simulink model "black_box"  (R2024b)
settings: Solver=ode1  StartTime=0.0  StopTime=Tobs  FixedStep=Ts  RelTol=1e-3
values from neighbouring files (symbols this model uses):
  delta_t = 10E-6    (= 1e-05)    [main_SVD.m]    (also in main_scan_FD.m)
  f0 = 50    [main_SVD.m]    (also in main_scan_FD.m)
  Id_ss = 0    [main_scan_FD.m]
  Ipeak = Sbase/Vpeak    [main_scan_FD.m]
  Iq_ss = 0    [main_scan_FD.m]
  P_finalvalue = 0.486    [main_scan_FD.m]    (also in main_ss_composite.m = 0.05)
  P_step_time = 1.5    [main_scan_FD.m]    (also in main_ss_composite.m = 10)
  phi = 0 * pi / 180    (= 0)    [main_SVD.m]
  signal_type = 1    [main_scan_FD.m]
  Ts = delta_t    (= 1e-05)    [main_scan_FD.m]
  V_finalvalue = 0.99    [main_ss_composite.m]
  V_step_time = 100    [main_scan_FD.m]    (also in main_ss_composite.m = 10)
  Vd_ss = 0    [main_scan_FD.m]
  Vpeak = (Vbase/sqrt(3))*sqrt(2)    [main_scan_FD.m]
  Vq_ss = 0    [main_scan_FD.m]
undefined symbols (not defined in the file or in its folder): C_dc, C_filt, dist_time, dist_value_0, dist_value_a, dist_value_b, dist_value_c, dist_value_d, dist_value_n, dist_value_p, dist_value_q, f_base, fd, I_charge, Iss_type, ki_inner_pu, ki_outer_P_pu, ki_outer_V_pu, ki_pll, kp_inner_pu, kp_outer_P_pu, kp_outer_V_pu, kp_pll, L, L_base, L_grid, L_vsc, omega_b, P_base, R_grid, R_vsc, Rsource, t_charge, V_base, V_dc, Vss_type
libraries: spsThreePhaseVIMeasurementLib x19, spsControlledVoltageSourceLib x15, spsControlledCurrentSourceLib x14, slpidlib x5, spsThreePhaseSeriesRLCBranchLib x4, spsabctodq0Lib x4, spsGroundLib x3, eeGeneralControl x1, spsLeadLagFilterLib x1, spsParallelRLCBranchLib x1, spsPLL3phLib x1, spsThreePhaseSourceLib x1
(part 3 of 3)

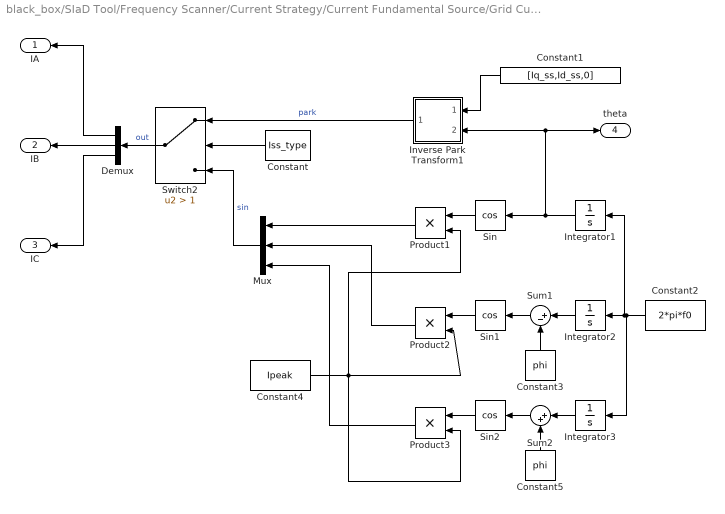
== system black_box/SIaD Tool/Frequency Scanner/Current Strategy/Current Fundamental Source/Grid Currents1 ==
  Constant : Constant  Value=Iss_type
  Constant1 : Constant  Value=[Iq_ss,Id_ss,0]  SampleTime=delta_t
  Constant2 : Constant  Value=2*pi*f0
  Constant3 : Constant  Value=phi
  Constant4 : Constant  Value=Ipeak
  Constant5 : Constant  Value=phi
  Demux : Demux  Outputs=3
  Integrator1 : Integrator  UpperSaturationLimit=1E100  LowerSaturationLimit=-1E100
  Integrator2 : Integrator  UpperSaturationLimit=1E100  LowerSaturationLimit=-1E100
  Integrator3 : Integrator  UpperSaturationLimit=1E100  LowerSaturationLimit=-1E100
  Inverse Park Transform1 : Subsystem
  Mux : Mux  Inputs=3
  Product1 : Product
  Product2 : Product
  Product3 : Product
  Sin : Trigonometry  Operator=cos
  Sin1 : Trigonometry  Operator=cos
  Sin2 : Trigonometry  Operator=cos
  Sum1 : Sum  Inputs=|+-
  Sum2 : Sum  Inputs=|++
  Switch2 : Switch  Criteria=u2 > Threshold  Threshold=1  SaturateOnIntegerOverflow=off  InputSameDT=off
  IA : Outport
  IB : Outport  Port=2
  IC : Outport  Port=3
  theta : Outport  Port=4
  wires:
  Constant1/1 -> Inverse Park Transform1/1(qd0)
  Demux/1 -> IA/1
  Demux/2 -> IB/1
  Demux/3 -> IC/1
  Product3/1 -> Mux/3
  Product1/1 -> Mux/1
  Sum1/1 -> Sin1/1
  Integrator2/1 -> Sum1/1
  Constant5/1 -> Sum2/2
  Integrator3/1 -> Sum2/1
  Sin/1 -> Product1/1
  Sin2/1 -> Product3/1
  Sin1/1 -> Product2/1
  Sum2/1 -> Sin2/1
  Constant2/1 -> Integrator1/1, Integrator2/1, Integrator3/1
  Integrator1/1 -> theta/1, Inverse Park Transform1/2(theta), Sin/1
  Constant4/1 -> Product2/2, Product1/2, Product3/2
  Product2/1 -> Mux/2
  Constant3/1 -> Sum1/2
  Switch2/1 -> Demux/1  "out"
  Inverse Park Transform1/1(ABC) -> Switch2/1  "park"
  Mux/1 -> Switch2/3  "sin"
  Constant/1 -> Switch2/2

== system black_box/SIaD Tool/Frequency Scanner/Current Strategy/pn0disturbance2/Multi-tone ==
  Clock : Clock
  Constant1 : Constant  Value=0
  From Workspace : FromWorkspace  VariableName=dist_value_0  SampleTime=delta_t  Interpolate=off  OutputAfterFinalValue=Holding final value
  From Workspace1 : FromWorkspace  VariableName=dist_value_p  SampleTime=delta_t  Interpolate=off  OutputAfterFinalValue=Holding final value
  From Workspace2 : FromWorkspace  VariableName=dist_value_n  SampleTime=delta_t  Interpolate=off  OutputAfterFinalValue=Holding final value
  Inverse Fortescue Transformation : Subsystem
  Mux : Mux  Inputs=3
  Switch1 : Switch  Criteria=u2 > Threshold  Threshold=dist_time  SaturateOnIntegerOverflow=off  InputSameDT=off
  Switch2 : Switch  Criteria=u2 > Threshold  Threshold=dist_time  SaturateOnIntegerOverflow=off  InputSameDT=off
  Switch3 : Switch  Criteria=u2 > Threshold  Threshold=dist_time  SaturateOnIntegerOverflow=off  InputSameDT=off
  ABC : Outport
  wires:
  Switch2/1 -> Mux/2
  From Workspace2/1 -> Switch3/1
  Constant1/1 -> Switch3/3, Switch2/3, Switch1/3
  From Workspace1/1 -> Switch2/1
  Switch3/1 -> Mux/3
  Clock/1 -> Switch1/2, Switch2/2, Switch3/2
  Switch1/1 -> Mux/1
  From Workspace/1 -> Switch1/1
  Mux/1 -> Inverse Fortescue Transformation/1(0PN)
  Inverse Fortescue Transformation/1(ABC) -> ABC/1

== system black_box/SIaD Tool/Frequency Scanner/Current Strategy/pn0disturbance2/Single-tone ==
  Constant1 : Constant  Value=2*pi*fd  SampleTime=delta_t
  Constant1111 : Constant  Value=0
  Constant222 : Constant  Value=dist_value_p
  Constant49 : Constant  Value=dist_value_0
  Constant50 : Constant  Value=dist_value_n
  Disturbance activator : Step  Time=dist_time  SampleTime=delta_t
  Integrator3 : Integrator
  Inverse Fortescue Transformation : Subsystem
  Math Function3 : Math
  Math Function4 : Math
  Math Function5 : Math
  Multiply2 : Gain
  Multiply3 : Gain
  Multiply4 : Gain
  Mux1 : Mux  Inputs=3
  Product{,4..5,8} (4 alike) : Product
  Real-Imag to Complex2 : RealImagToComplex
  Real-Imag to Complex3 : RealImagToComplex
  Real-Imag to Complex4 : RealImagToComplex
  ABC : Outport
  wires:
  Real-Imag to Complex3/1 -> Multiply2/1
  Math Function3/1 -> Product5/2
  Real-Imag to Complex2/1 -> Multiply3/1
  Inverse Fortescue Transformation/1(ABC) -> Product/2
  Disturbance activator/1 -> Product/1
  Product8/1 -> Mux1/2
  Integrator3/1 -> Real-Imag to Complex2/2, Real-Imag to Complex3/2, Real-Imag to Complex4/2
  Product/1 -> ABC/1
  Multiply2/1 -> Math Function4/1
  Real-Imag to Complex4/1 -> Multiply4/1
  Constant222/1 -> Product8/2
  Math Function5/1 -> Product4/2
  Constant49/1 -> Product4/1
  Mux1/1 -> Inverse Fortescue Transformation/1(0PN)
  Multiply3/1 -> Math Function3/1
  Multiply4/1 -> Math Function5/1
  Constant1/1 -> Integrator3/1
  Product4/1 -> Mux1/1
  Math Function4/1 -> Product8/1
  Constant1111/1 -> Real-Imag to Complex4/1, Real-Imag to Complex3/1, Real-Imag to Complex2/1
  Product5/1 -> Mux1/3
  Constant50/1 -> Product5/1

== system black_box/SIaD Tool/Frequency Scanner/Current Strategy/qd0disturbance2/Multi-tone ==
  In1 : Inport
  Clock1 : Clock
  Constant : Constant  Value=0
  From Workspace3 : FromWorkspace  VariableName=dist_value_q  SampleTime=delta_t  Interpolate=off  OutputAfterFinalValue=Holding final value
  From Workspace4 : FromWorkspace  VariableName=dist_value_d  SampleTime=delta_t  Interpolate=off  OutputAfterFinalValue=Holding final value
  Inverse Park Transform1 : Subsystem
  Mux3 : Mux  Inputs=3
  Switch : Switch  Criteria=u2 > Threshold  Threshold=dist_time  SaturateOnIntegerOverflow=off  InputSameDT=off
  Switch4 : Switch  Criteria=u2 > Threshold  Threshold=dist_time  SaturateOnIntegerOverflow=off  InputSameDT=off
  Vd : Constant  Value=0
  ABC : Outport
  wires:
  Inverse Park Transform1/1(ABC) -> ABC/1
  From Workspace3/1 -> Switch/1
  Clock1/1 -> Switch/2, Switch4/2
  Switch4/1 -> Mux3/2  "vd"
  Constant/1 -> Switch4/3, Switch/3
  Mux3/1 -> Inverse Park Transform1/1(qd0)
  Vd/1 -> Mux3/3
  From Workspace4/1 -> Switch4/1
  Switch/1 -> Mux3/1  "vq"
  In1/1 -> Inverse Park Transform1/2(theta)

== system black_box/SIaD Tool/Frequency Scanner/Current Strategy/qd0disturbance2/Single-tone ==
  note: qd disturbance
  In1 : Inport
  Constant18 : Constant  Value=dist_value_d
  Constant19 : Constant  Value=2*pi*fd
  Constant21 : Constant  Value=dist_value_q
  Cos : Trigonometry  Operator=cos
  Cos1 : Trigonometry  Operator=cos
  Disturbance activator : Step  Time=dist_time  Before=0.0  After=1.0  SampleTime=delta_t
  Integrator : Integrator
  Inverse Park Transform : Subsystem
  Mux23 : Mux  Inputs=3
  Product : Product
  Product4 : Product
  Product5 : Product
  V0 : Constant  Value=0
  ABC : Outport
  wires:
  Product/1 -> ABC/1
  Cos1/1 -> Product5/1
  Product4/1 -> Mux23/1
  Constant21/1 -> Product4/1
  Product5/1 -> Mux23/2
  Integrator/1 -> Cos/1, Cos1/1
  Cos/1 -> Product4/2
  Disturbance activator/1 -> Product/1
  Inverse Park Transform/1(ABC) -> Product/2
  Mux23/1 -> Inverse Park Transform/1(qd0)
  In1/1 -> Inverse Park Transform/2(theta)
  Constant18/1 -> Product5/2
  Constant19/1 -> Integrator/1
  V0/1 -> Mux23/3

== system black_box/SIaD Tool/Frequency Scanner/Voltage Strategy/ABCdisturbance/Multi-tone ==
  Clock : Clock
  Constant1 : Constant  Value=0
  From Workspace : FromWorkspace  VariableName=dist_value_a  SampleTime=delta_t  Interpolate=off  OutputAfterFinalValue=Holding final value
  From Workspace1 : FromWorkspace  VariableName=dist_value_b  SampleTime=delta_t  Interpolate=off  OutputAfterFinalValue=Holding final value
  From Workspace2 : FromWorkspace  VariableName=dist_value_c  SampleTime=delta_t  Interpolate=off  OutputAfterFinalValue=Holding final value
  Mux : Mux  Inputs=3
  Switch1 : Switch  Criteria=u2 > Threshold  Threshold=dist_time  SaturateOnIntegerOverflow=off  InputSameDT=off
  Switch2 : Switch  Criteria=u2 > Threshold  Threshold=dist_time  SaturateOnIntegerOverflow=off  InputSameDT=off
  Switch3 : Switch  Criteria=u2 > Threshold  Threshold=dist_time  SaturateOnIntegerOverflow=off  InputSameDT=off
  ABC : Outport
  wires:
  Switch2/1 -> Mux/2
  From Workspace2/1 -> Switch3/1
  Constant1/1 -> Switch3/3, Switch2/3, Switch1/3
  From Workspace1/1 -> Switch2/1
  Switch3/1 -> Mux/3
  Clock/1 -> Switch1/2, Switch2/2, Switch3/2
  Switch1/1 -> Mux/1
  From Workspace/1 -> Switch1/1
  Mux/1 -> ABC/1

== system black_box/SIaD Tool/Frequency Scanner/Voltage Strategy/ABCdisturbance/Single-tone ==
  note: ABC perturbance
  Constant10 : Constant  Value=phi
  Constant12 : Constant  Value=2*pi*fd  SampleTime=delta_t
  Constant9 : Constant  Value=phi
  Integrator5 : Integrator  UpperSaturationLimit=1E100  LowerSaturationLimit=-1E100
  Mux : Mux  Inputs=3
  Product1 : Product
  Product2 : Product
  Product3 : Product
  Sin : Trigonometry  Operator=cos
  Sin1 : Trigonometry  Operator=cos
  Sin2 : Trigonometry  Operator=cos
  Step1 : Step  Time=dist_time  After=dist_value_a  SampleTime=delta_t
  Step2 : Step  Time=dist_time  After=dist_value_b  SampleTime=delta_t
  Step3 : Step  Time=dist_time  After=dist_value_c  SampleTime=delta_t
  Sum6 : Sum  Inputs=|+-
  Sum7 : Sum  Inputs=|++
  ABC : Outport
  wires:
  Sin/1 -> Product1/1
  Sum7/1 -> Sin2/1
  Product1/1 -> Mux/1
  Integrator5/1 -> Sum7/1, Sin/1, Sum6/1
  Sin1/1 -> Product2/1
  Sin2/1 -> Product3/1
  Constant9/1 -> Sum6/2
  Constant10/1 -> Sum7/2
  Step3/1 -> Product3/2
  Step2/1 -> Product2/2
  Constant12/1 -> Integrator5/1
  Sum6/1 -> Sin1/1
  Step1/1 -> Product1/2
  Product2/1 -> Mux/2
  Product3/1 -> Mux/3
  Mux/1 -> ABC/1

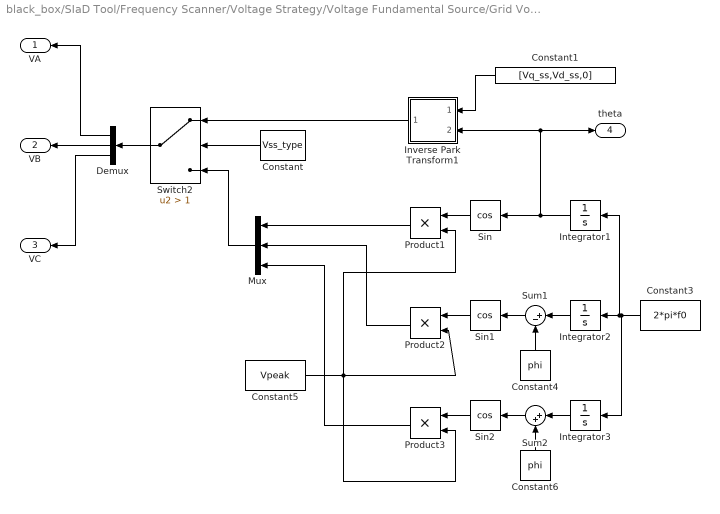
== system black_box/SIaD Tool/Frequency Scanner/Voltage Strategy/Voltage Fundamental Source/Grid Voltages ==
  Constant : Constant  Value=Vss_type
  Constant1 : Constant  Value=[Vq_ss,Vd_ss,0]  SampleTime=delta_t
  Constant3 : Constant  Value=2*pi*f0
  Constant4 : Constant  Value=phi
  Constant5 : Constant  Value=Vpeak
  Constant6 : Constant  Value=phi
  Demux : Demux  Outputs=3
  Integrator1 : Integrator  UpperSaturationLimit=1E100  LowerSaturationLimit=-1E100
  Integrator2 : Integrator  UpperSaturationLimit=1E100  LowerSaturationLimit=-1E100
  Integrator3 : Integrator  UpperSaturationLimit=1E100  LowerSaturationLimit=-1E100
  Inverse Park Transform1 : Subsystem
  Mux : Mux  Inputs=3
  Product1 : Product
  Product2 : Product
  Product3 : Product
  Sin : Trigonometry  Operator=cos
  Sin1 : Trigonometry  Operator=cos
  Sin2 : Trigonometry  Operator=cos
  Sum1 : Sum  Inputs=|+-
  Sum2 : Sum  Inputs=|++
  Switch2 : Switch  Criteria=u2 > Threshold  Threshold=1  SaturateOnIntegerOverflow=off  InputSameDT=off
  VA : Outport
  VB : Outport  Port=2
  VC : Outport  Port=3
  theta : Outport  Port=4
  wires:
  Demux/1 -> VA/1
  Demux/3 -> VC/1
  Demux/2 -> VB/1
  Constant5/1 -> Product2/2, Product1/2, Product3/2
  Mux/1 -> Switch2/3
  Product1/1 -> Mux/1
  Constant4/1 -> Sum1/2
  Integrator1/1 -> theta/1, Inverse Park Transform1/2(theta), Sin/1
  Product3/1 -> Mux/3
  Switch2/1 -> Demux/1
  Constant/1 -> Switch2/2
  Constant3/1 -> Integrator1/1, Integrator2/1, Integrator3/1
  Inverse Park Transform1/1(ABC) -> Switch2/1
  Sin1/1 -> Product2/1
  Integrator3/1 -> Sum2/1
  Integrator2/1 -> Sum1/1
  Sin2/1 -> Product3/1
  Constant1/1 -> Inverse Park Transform1/1(qd0)
  Sum2/1 -> Sin2/1
  Product2/1 -> Mux/2
  Constant6/1 -> Sum2/2
  Sin/1 -> Product1/1
  Sum1/1 -> Sin1/1

== system black_box/SIaD Tool/Frequency Scanner/Voltage Strategy/pn0disturbance/Multi-tone ==
  Clock : Clock
  Constant1 : Constant  Value=0
  From Workspace : FromWorkspace  VariableName=dist_value_0  SampleTime=delta_t  Interpolate=off  OutputAfterFinalValue=Holding final value
  From Workspace1 : FromWorkspace  VariableName=dist_value_p  SampleTime=delta_t  Interpolate=off  OutputAfterFinalValue=Holding final value
  From Workspace2 : FromWorkspace  VariableName=dist_value_n  SampleTime=delta_t  Interpolate=off  OutputAfterFinalValue=Holding final value
  Inverse Fortescue Transformation : Subsystem
  Mux : Mux  Inputs=3
  Switch1 : Switch  Criteria=u2 > Threshold  Threshold=dist_time  SaturateOnIntegerOverflow=off  InputSameDT=off
  Switch2 : Switch  Criteria=u2 > Threshold  Threshold=dist_time  SaturateOnIntegerOverflow=off  InputSameDT=off
  Switch3 : Switch  Criteria=u2 > Threshold  Threshold=dist_time  SaturateOnIntegerOverflow=off  InputSameDT=off
  ABC : Outport
  wires:
  Switch2/1 -> Mux/2
  From Workspace2/1 -> Switch3/1
  Constant1/1 -> Switch3/3, Switch2/3, Switch1/3
  From Workspace1/1 -> Switch2/1
  Switch3/1 -> Mux/3
  Clock/1 -> Switch1/2, Switch2/2, Switch3/2
  Switch1/1 -> Mux/1
  From Workspace/1 -> Switch1/1
  Mux/1 -> Inverse Fortescue Transformation/1(0PN)
  Inverse Fortescue Transformation/1(ABC) -> ABC/1

== system black_box/SIaD Tool/Frequency Scanner/Voltage Strategy/pn0disturbance/Single-tone ==
  Constant1 : Constant  Value=2*pi*fd  SampleTime=delta_t
  Constant1111 : Constant  Value=0
  Constant222 : Constant  Value=dist_value_p
  Constant49 : Constant  Value=dist_value_0
  Constant50 : Constant  Value=dist_value_n
  Disturbance activator : Step  Time=dist_time  SampleTime=delta_t
  Integrator3 : Integrator
  Inverse Fortescue Transformation : Subsystem
  Math Function3 : Math
  Math Function4 : Math
  Math Function5 : Math
  Multiply2 : Gain
  Multiply3 : Gain
  Multiply4 : Gain
  Mux1 : Mux  Inputs=3
  Product{,4..5,8} (4 alike) : Product
  Real-Imag to Complex2 : RealImagToComplex
  Real-Imag to Complex3 : RealImagToComplex
  Real-Imag to Complex4 : RealImagToComplex
  ABC : Outport
  wires:
  Real-Imag to Complex3/1 -> Multiply2/1
  Math Function3/1 -> Product5/2
  Real-Imag to Complex2/1 -> Multiply3/1
  Inverse Fortescue Transformation/1(ABC) -> Product/2
  Disturbance activator/1 -> Product/1
  Product8/1 -> Mux1/2
  Integrator3/1 -> Real-Imag to Complex2/2, Real-Imag to Complex3/2, Real-Imag to Complex4/2
  Product/1 -> ABC/1
  Multiply2/1 -> Math Function4/1
  Real-Imag to Complex4/1 -> Multiply4/1
  Constant222/1 -> Product8/2
  Math Function5/1 -> Product4/2
  Constant49/1 -> Product4/1
  Mux1/1 -> Inverse Fortescue Transformation/1(0PN)
  Multiply3/1 -> Math Function3/1
  Multiply4/1 -> Math Function5/1
  Constant1/1 -> Integrator3/1
  Product4/1 -> Mux1/1
  Math Function4/1 -> Product8/1
  Constant1111/1 -> Real-Imag to Complex4/1, Real-Imag to Complex3/1, Real-Imag to Complex2/1
  Product5/1 -> Mux1/3
  Constant50/1 -> Product5/1

== system black_box/SIaD Tool/Frequency Scanner/Voltage Strategy/qd0disturbance/Multi-tone ==
  In1 : Inport
  Clock1 : Clock
  Constant : Constant  Value=0
  From Workspace3 : FromWorkspace  VariableName=dist_value_q  SampleTime=delta_t  Interpolate=off  OutputAfterFinalValue=Holding final value
  From Workspace4 : FromWorkspace  VariableName=dist_value_d  SampleTime=delta_t  Interpolate=off  OutputAfterFinalValue=Holding final value
  Inverse Park Transform1 : Subsystem
  Mux3 : Mux  Inputs=3
  Switch : Switch  Criteria=u2 > Threshold  Threshold=dist_time  SaturateOnIntegerOverflow=off  InputSameDT=off
  Switch4 : Switch  Criteria=u2 > Threshold  Threshold=dist_time  SaturateOnIntegerOverflow=off  InputSameDT=off
  Vd : Constant  Value=0
  ABC : Outport
  wires:
  Inverse Park Transform1/1(ABC) -> ABC/1
  From Workspace3/1 -> Switch/1
  Clock1/1 -> Switch/2, Switch4/2
  Switch4/1 -> Mux3/2  "vd"
  Constant/1 -> Switch4/3, Switch/3
  Mux3/1 -> Inverse Park Transform1/1(qd0)
  Vd/1 -> Mux3/3
  From Workspace4/1 -> Switch4/1
  Switch/1 -> Mux3/1  "vq"
  In1/1 -> Inverse Park Transform1/2(theta)

== system black_box/SIaD Tool/Frequency Scanner/Voltage Strategy/qd0disturbance/Single-tone ==
  note: qd disturbance
  In1 : Inport
  Constant18 : Constant  Value=dist_value_d
  Constant19 : Constant  Value=2*pi*fd
  Constant21 : Constant  Value=dist_value_q
  Cos : Trigonometry  Operator=cos
  Cos1 : Trigonometry  Operator=cos
  Disturbance activator : Step  Time=dist_time  Before=0.0  After=1.0  SampleTime=delta_t
  Integrator : Integrator
  Inverse Park Transform : Subsystem
  Mux23 : Mux  Inputs=3
  Product : Product
  Product4 : Product
  Product5 : Product
  V0 : Constant  Value=0
  ABC : Outport
  wires:
  Product/1 -> ABC/1
  Cos1/1 -> Product5/1
  Product4/1 -> Mux23/1
  Constant21/1 -> Product4/1
  Product5/1 -> Mux23/2
  Integrator/1 -> Cos/1, Cos1/1
  Cos/1 -> Product4/2
  Disturbance activator/1 -> Product/1
  Inverse Park Transform/1(ABC) -> Product/2
  Mux23/1 -> Inverse Park Transform/1(qd0)
  In1/1 -> Inverse Park Transform/2(theta)
  Constant18/1 -> Product5/2
  Constant19/1 -> Integrator/1
  V0/1 -> Mux23/3

== system black_box/SIaD Tool/Frequency Scanner/Current Strategy/Current Fundamental Source/Grid Currents1/Inverse Park Transform1 ==
  qd0 : Inport
  theta : Inport  Port=2
  Constant : Constant
  Constant3 : Constant  Value=(2*pi)/3
  Constant4 : Constant  Value=(2*pi)/3
  Cos : Trigonometry  Operator=cos
  Matrix Concatenate : Concatenate  NumInputs=3  Mode=Multidimensional array  ConcatenateDimension=2
  Matrix Multiply : Product  Multiplication=Matrix(*)
  Mux : Mux  Inputs=3
  Mux1 : Mux  Inputs=3
  Sin : Trigonometry
  Sum : Sum  Inputs=+-
  Sum1 : Sum  Inputs=|++
  ABC : Outport
  wires:
  Constant3/1 -> Sum/2
  Constant4/1 -> Sum1/2
  qd0/1 -> Matrix Multiply/2
  Matrix Multiply/1 -> ABC/1
  theta/1 -> Sum1/1, Sum/1, Mux/1
  Sum/1 -> Mux/2
  Sum1/1 -> Mux/3
  Mux/1 -> Sin/1, Cos/1
  Cos/1 -> Matrix Concatenate/1
  Sin/1 -> Matrix Concatenate/2
  Constant/1 -> Mux1/3, Mux1/1, Mux1/2
  Mux1/1 -> Matrix Concatenate/3
  Matrix Concatenate/1 -> Matrix Multiply/1

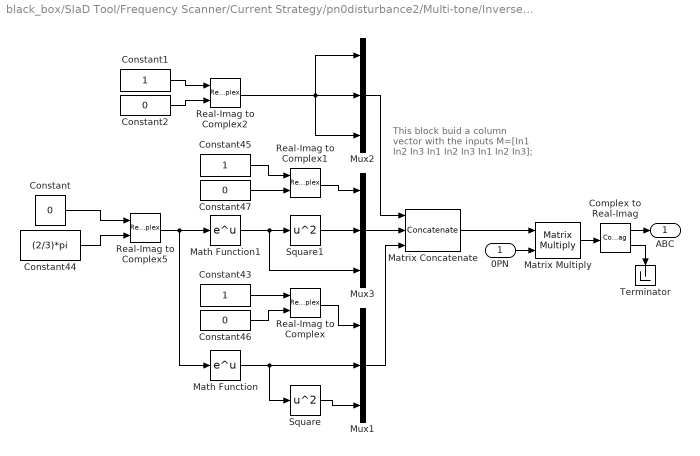
== system black_box/SIaD Tool/Frequency Scanner/Current Strategy/pn0disturbance2/Multi-tone/Inverse Fortescue Transformation ==
  note: This block buid a column vector with the inputs
      | M=[In1 In2 In3
      |       In1 In2 In3
      |       In1 In2 In3];
  0PN : Inport
  Complex to Real-Imag : ComplexToRealImag
  Constant{,2,46..47} (4 alike) : Constant  Value=0
  Constant1 : Constant
  Constant43 : Constant
  Constant44 : Constant  Value=(2/3)*pi
  Constant45 : Constant
  Math Function : Math
  Math Function1 : Math
  Matrix Concatenate : Concatenate  NumInputs=3  Mode=Multidimensional array  ConcatenateDimension=2
  Matrix Multiply : Product  Multiplication=Matrix(*)
  Mux1 : Mux  Inputs=3
  Mux2 : Mux  Inputs=3
  Mux3 : Mux  Inputs=3
  Real-Imag to Complex{,1..2,5} (4 alike) : RealImagToComplex
  Square : Math  Operator=square
  Square1 : Math  Operator=square
  Terminator : Terminator
  ABC : Outport
  wires:
  Real-Imag to Complex5/1 -> Math Function/1, Math Function1/1
  Constant45/1 -> Real-Imag to Complex1/1
  Constant46/1 -> Real-Imag to Complex/2
  Constant43/1 -> Real-Imag to Complex/1
  Math Function/1 -> Mux1/2, Square/1
  Matrix Concatenate/1 -> Matrix Multiply/1
  Square1/1 -> Mux3/2
  Real-Imag to Complex2/1 -> Mux2/2, Mux2/1, Mux2/3
  0PN/1 -> Matrix Multiply/2
  Math Function1/1 -> Square1/1, Mux3/3
  Constant47/1 -> Real-Imag to Complex1/2
  Mux1/1 -> Matrix Concatenate/3
  Mux2/1 -> Matrix Concatenate/1
  Square/1 -> Mux1/3
  Real-Imag to Complex/1 -> Mux1/1
  Real-Imag to Complex1/1 -> Mux3/1
  Mux3/1 -> Matrix Concatenate/2
  Matrix Multiply/1 -> Complex to Real-Imag/1
  Complex to Real-Imag/1 -> ABC/1
  Complex to Real-Imag/2 -> Terminator/1
  Constant44/1 -> Real-Imag to Complex5/2
  Constant/1 -> Real-Imag to Complex5/1
  Constant2/1 -> Real-Imag to Complex2/2
  Constant1/1 -> Real-Imag to Complex2/1

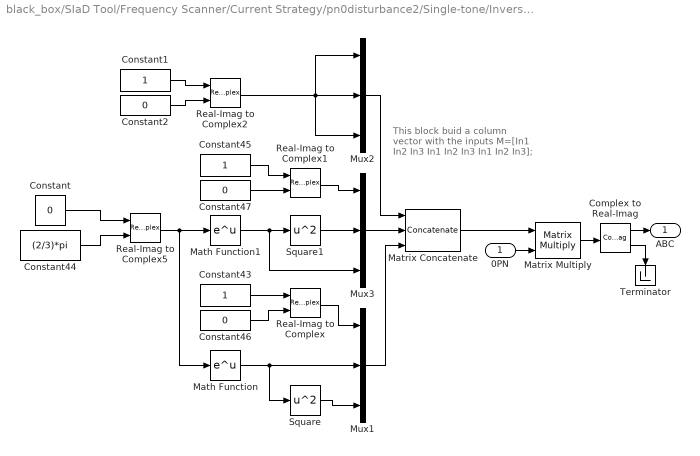
== system black_box/SIaD Tool/Frequency Scanner/Current Strategy/pn0disturbance2/Single-tone/Inverse Fortescue Transformation ==
  note: This block buid a column vector with the inputs
      | M=[In1 In2 In3
      |       In1 In2 In3
      |       In1 In2 In3];
  0PN : Inport
  Complex to Real-Imag : ComplexToRealImag
  Constant{,2,46..47} (4 alike) : Constant  Value=0
  Constant1 : Constant
  Constant43 : Constant
  Constant44 : Constant  Value=(2/3)*pi
  Constant45 : Constant
  Math Function : Math
  Math Function1 : Math
  Matrix Concatenate : Concatenate  NumInputs=3  Mode=Multidimensional array  ConcatenateDimension=2
  Matrix Multiply : Product  Multiplication=Matrix(*)
  Mux1 : Mux  Inputs=3
  Mux2 : Mux  Inputs=3
  Mux3 : Mux  Inputs=3
  Real-Imag to Complex{,1..2,5} (4 alike) : RealImagToComplex
  Square : Math  Operator=square
  Square1 : Math  Operator=square
  Terminator : Terminator
  ABC : Outport
  wires:
  Real-Imag to Complex5/1 -> Math Function/1, Math Function1/1
  Constant45/1 -> Real-Imag to Complex1/1
  Constant46/1 -> Real-Imag to Complex/2
  Constant43/1 -> Real-Imag to Complex/1
  Math Function/1 -> Mux1/2, Square/1
  Matrix Concatenate/1 -> Matrix Multiply/1
  Square1/1 -> Mux3/2
  Real-Imag to Complex2/1 -> Mux2/2, Mux2/1, Mux2/3
  0PN/1 -> Matrix Multiply/2
  Math Function1/1 -> Square1/1, Mux3/3
  Constant47/1 -> Real-Imag to Complex1/2
  Mux1/1 -> Matrix Concatenate/3
  Mux2/1 -> Matrix Concatenate/1
  Square/1 -> Mux1/3
  Real-Imag to Complex/1 -> Mux1/1
  Real-Imag to Complex1/1 -> Mux3/1
  Mux3/1 -> Matrix Concatenate/2
  Matrix Multiply/1 -> Complex to Real-Imag/1
  Complex to Real-Imag/1 -> ABC/1
  Complex to Real-Imag/2 -> Terminator/1
  Constant44/1 -> Real-Imag to Complex5/2
  Constant/1 -> Real-Imag to Complex5/1
  Constant2/1 -> Real-Imag to Complex2/2
  Constant1/1 -> Real-Imag to Complex2/1

== system black_box/SIaD Tool/Frequency Scanner/Current Strategy/qd0disturbance2/Multi-tone/Inverse Park Transform1 ==
  qd0 : Inport
  theta : Inport  Port=2
  Constant : Constant
  Constant3 : Constant  Value=(2*pi)/3
  Constant4 : Constant  Value=(2*pi)/3
  Cos : Trigonometry  Operator=cos
  Matrix Concatenate : Concatenate  NumInputs=3  Mode=Multidimensional array  ConcatenateDimension=2
  Matrix Multiply : Product  Multiplication=Matrix(*)
  Mux : Mux  Inputs=3
  Mux1 : Mux  Inputs=3
  Sin : Trigonometry
  Sum : Sum  Inputs=+-
  Sum1 : Sum  Inputs=|++
  ABC : Outport
  wires:
  Constant3/1 -> Sum/2
  Constant4/1 -> Sum1/2
  qd0/1 -> Matrix Multiply/2
  Matrix Multiply/1 -> ABC/1
  theta/1 -> Sum1/1, Sum/1, Mux/1
  Sum/1 -> Mux/2
  Sum1/1 -> Mux/3
  Mux/1 -> Sin/1, Cos/1
  Cos/1 -> Matrix Concatenate/1
  Sin/1 -> Matrix Concatenate/2
  Constant/1 -> Mux1/3, Mux1/1, Mux1/2
  Mux1/1 -> Matrix Concatenate/3
  Matrix Concatenate/1 -> Matrix Multiply/1

== system black_box/SIaD Tool/Frequency Scanner/Current Strategy/qd0disturbance2/Single-tone/Inverse Park Transform ==
  qd0 : Inport
  theta : Inport  Port=2
  Constant : Constant
  Constant3 : Constant  Value=(2*pi)/3
  Constant4 : Constant  Value=(2*pi)/3
  Cos : Trigonometry  Operator=cos
  Matrix Concatenate : Concatenate  NumInputs=3  Mode=Multidimensional array  ConcatenateDimension=2
  Matrix Multiply : Product  Multiplication=Matrix(*)
  Mux : Mux  Inputs=3
  Mux1 : Mux  Inputs=3
  Sin : Trigonometry
  Sum : Sum  Inputs=+-
  Sum1 : Sum  Inputs=|++
  ABC : Outport
  wires:
  Constant3/1 -> Sum/2
  Constant4/1 -> Sum1/2
  qd0/1 -> Matrix Multiply/2
  Matrix Multiply/1 -> ABC/1
  theta/1 -> Sum1/1, Sum/1, Mux/1
  Sum/1 -> Mux/2
  Sum1/1 -> Mux/3
  Mux/1 -> Sin/1, Cos/1
  Cos/1 -> Matrix Concatenate/1
  Sin/1 -> Matrix Concatenate/2
  Constant/1 -> Mux1/3, Mux1/1, Mux1/2
  Mux1/1 -> Matrix Concatenate/3
  Matrix Concatenate/1 -> Matrix Multiply/1

== system black_box/SIaD Tool/Frequency Scanner/Voltage Strategy/Voltage Fundamental Source/Grid Voltages/Inverse Park Transform1 ==
  qd0 : Inport
  theta : Inport  Port=2
  Constant : Constant
  Constant3 : Constant  Value=(2*pi)/3
  Constant4 : Constant  Value=(2*pi)/3
  Cos : Trigonometry  Operator=cos
  Matrix Concatenate : Concatenate  NumInputs=3  Mode=Multidimensional array  ConcatenateDimension=2
  Matrix Multiply : Product  Multiplication=Matrix(*)
  Mux : Mux  Inputs=3
  Mux1 : Mux  Inputs=3
  Sin : Trigonometry
  Sum : Sum  Inputs=+-
  Sum1 : Sum  Inputs=|++
  ABC : Outport
  wires:
  Constant3/1 -> Sum/2
  Constant4/1 -> Sum1/2
  qd0/1 -> Matrix Multiply/2
  Matrix Multiply/1 -> ABC/1
  theta/1 -> Sum1/1, Sum/1, Mux/1
  Sum/1 -> Mux/2
  Sum1/1 -> Mux/3
  Mux/1 -> Sin/1, Cos/1
  Cos/1 -> Matrix Concatenate/1
  Sin/1 -> Matrix Concatenate/2
  Constant/1 -> Mux1/3, Mux1/1, Mux1/2
  Mux1/1 -> Matrix Concatenate/3
  Matrix Concatenate/1 -> Matrix Multiply/1

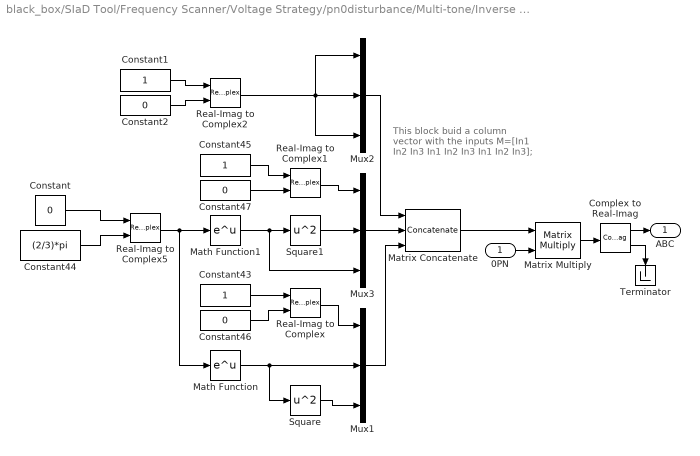
== system black_box/SIaD Tool/Frequency Scanner/Voltage Strategy/pn0disturbance/Multi-tone/Inverse Fortescue Transformation ==
  note: This block buid a column vector with the inputs
      | M=[In1 In2 In3
      |       In1 In2 In3
      |       In1 In2 In3];
  0PN : Inport
  Complex to Real-Imag : ComplexToRealImag
  Constant{,2,46..47} (4 alike) : Constant  Value=0
  Constant1 : Constant
  Constant43 : Constant
  Constant44 : Constant  Value=(2/3)*pi
  Constant45 : Constant
  Math Function : Math
  Math Function1 : Math
  Matrix Concatenate : Concatenate  NumInputs=3  Mode=Multidimensional array  ConcatenateDimension=2
  Matrix Multiply : Product  Multiplication=Matrix(*)
  Mux1 : Mux  Inputs=3
  Mux2 : Mux  Inputs=3
  Mux3 : Mux  Inputs=3
  Real-Imag to Complex{,1..2,5} (4 alike) : RealImagToComplex
  Square : Math  Operator=square
  Square1 : Math  Operator=square
  Terminator : Terminator
  ABC : Outport
  wires:
  Real-Imag to Complex5/1 -> Math Function/1, Math Function1/1
  Constant45/1 -> Real-Imag to Complex1/1
  Constant46/1 -> Real-Imag to Complex/2
  Constant43/1 -> Real-Imag to Complex/1
  Math Function/1 -> Mux1/2, Square/1
  Matrix Concatenate/1 -> Matrix Multiply/1
  Square1/1 -> Mux3/2
  Real-Imag to Complex2/1 -> Mux2/2, Mux2/1, Mux2/3
  0PN/1 -> Matrix Multiply/2
  Math Function1/1 -> Square1/1, Mux3/3
  Constant47/1 -> Real-Imag to Complex1/2
  Mux1/1 -> Matrix Concatenate/3
  Mux2/1 -> Matrix Concatenate/1
  Square/1 -> Mux1/3
  Real-Imag to Complex/1 -> Mux1/1
  Real-Imag to Complex1/1 -> Mux3/1
  Mux3/1 -> Matrix Concatenate/2
  Matrix Multiply/1 -> Complex to Real-Imag/1
  Complex to Real-Imag/1 -> ABC/1
  Complex to Real-Imag/2 -> Terminator/1
  Constant44/1 -> Real-Imag to Complex5/2
  Constant/1 -> Real-Imag to Complex5/1
  Constant2/1 -> Real-Imag to Complex2/2
  Constant1/1 -> Real-Imag to Complex2/1

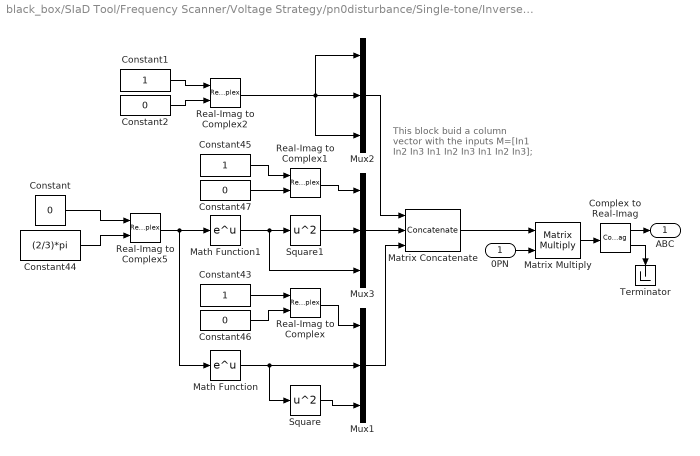
== system black_box/SIaD Tool/Frequency Scanner/Voltage Strategy/pn0disturbance/Single-tone/Inverse Fortescue Transformation ==
  note: This block buid a column vector with the inputs
      | M=[In1 In2 In3
      |       In1 In2 In3
      |       In1 In2 In3];
  0PN : Inport
  Complex to Real-Imag : ComplexToRealImag
  Constant{,2,46..47} (4 alike) : Constant  Value=0
  Constant1 : Constant
  Constant43 : Constant
  Constant44 : Constant  Value=(2/3)*pi
  Constant45 : Constant
  Math Function : Math
  Math Function1 : Math
  Matrix Concatenate : Concatenate  NumInputs=3  Mode=Multidimensional array  ConcatenateDimension=2
  Matrix Multiply : Product  Multiplication=Matrix(*)
  Mux1 : Mux  Inputs=3
  Mux2 : Mux  Inputs=3
  Mux3 : Mux  Inputs=3
  Real-Imag to Complex{,1..2,5} (4 alike) : RealImagToComplex
  Square : Math  Operator=square
  Square1 : Math  Operator=square
  Terminator : Terminator
  ABC : Outport
  wires:
  Real-Imag to Complex5/1 -> Math Function/1, Math Function1/1
  Constant45/1 -> Real-Imag to Complex1/1
  Constant46/1 -> Real-Imag to Complex/2
  Constant43/1 -> Real-Imag to Complex/1
  Math Function/1 -> Mux1/2, Square/1
  Matrix Concatenate/1 -> Matrix Multiply/1
  Square1/1 -> Mux3/2
  Real-Imag to Complex2/1 -> Mux2/2, Mux2/1, Mux2/3
  0PN/1 -> Matrix Multiply/2
  Math Function1/1 -> Square1/1, Mux3/3
  Constant47/1 -> Real-Imag to Complex1/2
  Mux1/1 -> Matrix Concatenate/3
  Mux2/1 -> Matrix Concatenate/1
  Square/1 -> Mux1/3
  Real-Imag to Complex/1 -> Mux1/1
  Real-Imag to Complex1/1 -> Mux3/1
  Mux3/1 -> Matrix Concatenate/2
  Matrix Multiply/1 -> Complex to Real-Imag/1
  Complex to Real-Imag/1 -> ABC/1
  Complex to Real-Imag/2 -> Terminator/1
  Constant44/1 -> Real-Imag to Complex5/2
  Constant/1 -> Real-Imag to Complex5/1
  Constant2/1 -> Real-Imag to Complex2/2
  Constant1/1 -> Real-Imag to Complex2/1

== system black_box/SIaD Tool/Frequency Scanner/Voltage Strategy/qd0disturbance/Multi-tone/Inverse Park Transform1 ==
  qd0 : Inport
  theta : Inport  Port=2
  Constant : Constant
  Constant3 : Constant  Value=(2*pi)/3
  Constant4 : Constant  Value=(2*pi)/3
  Cos : Trigonometry  Operator=cos
  Matrix Concatenate : Concatenate  NumInputs=3  Mode=Multidimensional array  ConcatenateDimension=2
  Matrix Multiply : Product  Multiplication=Matrix(*)
  Mux : Mux  Inputs=3
  Mux1 : Mux  Inputs=3
  Sin : Trigonometry
  Sum : Sum  Inputs=+-
  Sum1 : Sum  Inputs=|++
  ABC : Outport
  wires:
  Constant3/1 -> Sum/2
  Constant4/1 -> Sum1/2
  qd0/1 -> Matrix Multiply/2
  Matrix Multiply/1 -> ABC/1
  theta/1 -> Sum1/1, Sum/1, Mux/1
  Sum/1 -> Mux/2
  Sum1/1 -> Mux/3
  Mux/1 -> Sin/1, Cos/1
  Cos/1 -> Matrix Concatenate/1
  Sin/1 -> Matrix Concatenate/2
  Constant/1 -> Mux1/3, Mux1/1, Mux1/2
  Mux1/1 -> Matrix Concatenate/3
  Matrix Concatenate/1 -> Matrix Multiply/1

== system black_box/SIaD Tool/Frequency Scanner/Voltage Strategy/qd0disturbance/Single-tone/Inverse Park Transform ==
  qd0 : Inport
  theta : Inport  Port=2
  Constant : Constant
  Constant3 : Constant  Value=(2*pi)/3
  Constant4 : Constant  Value=(2*pi)/3
  Cos : Trigonometry  Operator=cos
  Matrix Concatenate : Concatenate  NumInputs=3  Mode=Multidimensional array  ConcatenateDimension=2
  Matrix Multiply : Product  Multiplication=Matrix(*)
  Mux : Mux  Inputs=3
  Mux1 : Mux  Inputs=3
  Sin : Trigonometry
  Sum : Sum  Inputs=+-
  Sum1 : Sum  Inputs=|++
  ABC : Outport
  wires:
  Constant3/1 -> Sum/2
  Constant4/1 -> Sum1/2
  qd0/1 -> Matrix Multiply/2
  Matrix Multiply/1 -> ABC/1
  theta/1 -> Sum1/1, Sum/1, Mux/1
  Sum/1 -> Mux/2
  Sum1/1 -> Mux/3
  Mux/1 -> Sin/1, Cos/1
  Cos/1 -> Matrix Concatenate/1
  Sin/1 -> Matrix Concatenate/2
  Constant/1 -> Mux1/3, Mux1/1, Mux1/2
  Mux1/1 -> Matrix Concatenate/3
  Matrix Concatenate/1 -> Matrix Multiply/1
